simulink model "geki_Jin"  (Simulink 8.7)
settings: Solver=FixedStepDiscrete  StartTime=0.0  StopTime=1  FixedStep=1e-2  RelTol=1e-3
StopFcn:
  | t;
  | t11;
  | t2;
  | t31;
  | t41;
undefined symbols (not defined in the file or in its folder): DiscIntNeverNeededParam
settings Model: Creator=Administrator  LastModifiedBy=ACER
settings DataIOCC: SignalLoggingSaveFormat=ModelDataLogs  SaveOutput=off  SignalLogging=off  DSMLogging=off  SaveTime=off
settings OptimizationCC: ExpressionDepthLimit=2147483647
settings DebuggingCC: FcnCallInpInsideContextMsg=EnableAllAsWarning  StateNameClashWarn=warning
settings ConfigComp: CovSFcnEnable=off

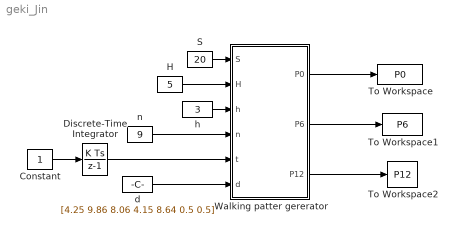
== system geki_Jin ==
  Constant : Constant
  Discrete-Time Integrator : DiscreteIntegrator  SampleTime=1e-2  ICPrevOutput=DiscIntNeverNeededParam  ICPrevScaledInput=DiscIntNeverNeededParam
  H : Constant  Value=5
  S : Constant  Value=20
  To Workspace : ToWorkspace  VariableName=P0  SampleTime=-1
      settings: Save2DSignal=2-D array (concatenate along first dimension)
  To Workspace1 : ToWorkspace  VariableName=P6  SampleTime=-1
      settings: Save2DSignal=2-D array (concatenate along first dimension)
  To Workspace2 : ToWorkspace  VariableName=P12  SampleTime=-1
      settings: Save2DSignal=2-D array (concatenate along first dimension)
  Walking patter gererator : MATLAB Function  TreatAsAtomicUnit=on
  d : Constant  Value=[4.25 9.86 8.06 4.15 8.64 0.5 0.5]
  h : Constant  Value=3
  n : Constant  Value=9
  wires:
  Walking patter gererator/3(P12) -> To Workspace2/1
  Walking patter gererator/2(P6) -> To Workspace1/1
  h/1 -> Walking patter gererator/3(h)
  d/1 -> Walking patter gererator/6(d)
  Constant/1 -> Discrete-Time Integrator/1
  Discrete-Time Integrator/1 -> Walking patter gererator/5(t)
  S/1 -> Walking patter gererator/1(S)
  H/1 -> Walking patter gererator/2(H)
  n/1 -> Walking patter gererator/4(n)
  Walking patter gererator/1(P0) -> To Workspace/1

== matlab function Walking patter gererator ==
  data: S input double; H input double; h input double; n input double; P0 output double; P6 output double; P12 output double; t input double; d input double
function [P0, P6, P12] = fcn(S, H,h, n, t, d)
d1 = d(1);
d2 = d(2);
d3 = d(3);
d4 = d(4);
W = d(5);
t1=d(6);
t2=d(7);
T=1;
t0=0;
% P0x
    if t>=T
        P0x= -(S/2)*sin((pi/T)*(t-T/2));
    else
        P0x=0;
    end
% Poy
    if t>=T
        P0y=W;
    else
        P0y=0;
    end
% P0z
    if t>=T
        P0z=H*sin(pi*(P0x/S+0.5));
    else
        P0z=0;
    end
% P12x
    if t<T
        P12x=(S/2)*sin((pi/T)*(t-T/2));
    else
        P12x=0;
    end
% P12y
    if t<T
        P12y=-W;
    else
        P12y=0;
    end
  
% P12z
   if t<T     
        P12z=H*sin(pi*(P12x/S+0.5));
   else
        P12z=0;
   end
% P6x
   if t<=T
     t0=t;
   end
   if t>T
     t0=t-T;
   end
   P6x=(S/4)*sin((pi/T)*(t0-T/2));
% P6y
%    if t<=T
%      t1=t;
%    end
%    if t>T
%      t1=t-T;
%    end
%    P6y=n*sin((pi/2)*(sin((t1*pi)/(2*T))+1))*sin(pi*t/T);

P6y=n*sin(pi/(2*t1)*t)*(u(t)-u(t-t1))...
             +n*(u(t-t1)-u(t-t2))...
             +n*cos(pi/(2*(T-t2))*(t-t2))*(u(t-t2)-u(t-T));
% P6z
   P6z=d1+d2+d3+d4-h;
P0 = [P0x,P0y,P0z];
P6 = [P6x,P6y,P6z];
P12 = [P12x,P12y,P12z];
end
function ti=u(t)
    if (t>=0)
        ti=1;
    else
        ti=0;
    end
end
